simulink model "controller"  (R2018b)
settings: Solver=FixedStepAuto  StartTime=0.0  StopTime=15  FixedStep=0.005  RelTol=1e-3
settings Model: NumberOfSteps=50  Creator=XLIYAN  LastModifiedBy=XLIYAN
settings DebuggingCC: VectorMatrixConversionMsg=warning  UnderSpecifiedDimensionMsg=warning

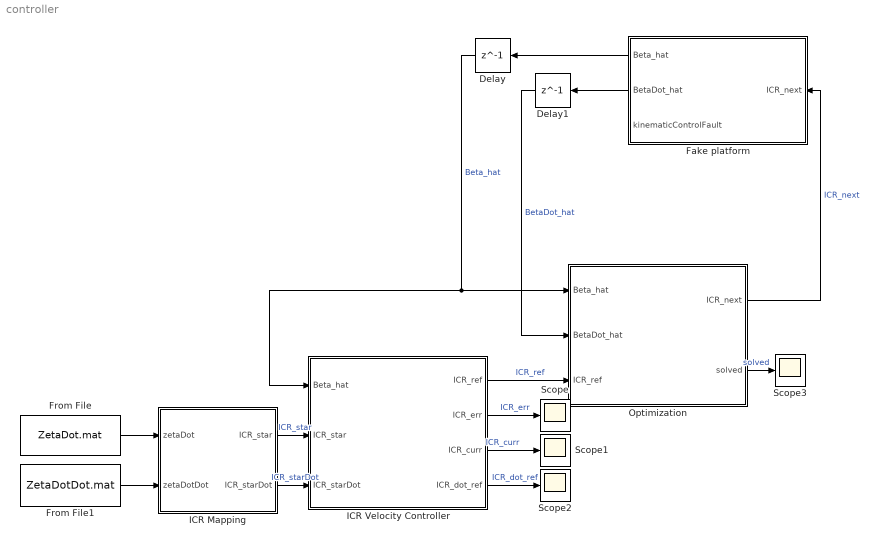
== system controller ==
  Delay : Delay  DelayLength=1  InitialCondition=[0,0,0,0]  InputProcessing=Inherited  SampleTime=0.005
  Delay1 : Delay  DelayLength=1  InitialCondition=[0,0,0,0]  InputProcessing=Inherited  SampleTime=0.005
  Fake platform : MATLAB Function  TreatAsAtomicUnit=on
  From File : FromFile  FileName=ZetaDot.mat  SampleTime=0
  From File1 : FromFile  FileName=ZetaDotDot.mat  SampleTime=0
  ICR Mapping : MATLAB Function  TreatAsAtomicUnit=on
  ICR Velocity Controller : MATLAB Function  TreatAsAtomicUnit=on
  Optimization : MATLAB Function  TreatAsAtomicUnit=on
  Scope{,1..3} (4 alike) : Scope
  wires:
  From File/1 -> ICR Mapping/1(zetaDot)
  From File1/1 -> ICR Mapping/2(zetaDotDot)
  ICR Mapping/1(ICR_star) -> ICR Velocity Controller/2(ICR_star)  "ICR_star"
  ICR Mapping/2(ICR_starDot) -> ICR Velocity Controller/3(ICR_starDot)  "ICR_starDot"
  ICR Velocity Controller/1(ICR_ref) -> Optimization/3(ICR_ref)  "ICR_ref"
  Fake platform/1(Beta_hat) -> Delay/1
  Delay/1 -> ICR Velocity Controller/1(Beta_hat), Optimization/1(Beta_hat)  "Beta_hat"
  Fake platform/2(BetaDot_hat) -> Delay1/1
  Delay1/1 -> Optimization/2(BetaDot_hat)  "BetaDot_hat"
  Optimization/1(ICR_next) -> Fake platform/1(ICR_next)  "ICR_next"
  ICR Velocity Controller/2(ICR_err) -> Scope/1  "ICR_err"
  ICR Velocity Controller/3(ICR_curr) -> Scope1/1  "ICR_curr"
  ICR Velocity Controller/4(ICR_dot_ref) -> Scope2/1  "ICR_dot_ref"
  Optimization/2(solved) -> Scope3/1  "solved"

== matlab function controller/ICR Velocity Controller ==
  data: Beta_hat input; ICR_star input; ICR_ref output; ICR_starDot input; ICR_err output; ICR_curr output; ICR_dot_ref output
function [ICR_ref,ICR_err,ICR_curr,ICR_dot_ref] = ICR_vel_Controller(Beta_hat, ICR_star, ICR_starDot)

vehicle.length = 0.526;  % Vehicle length
vehicle.width = 0.526;   % Vehicle width
wheel.radius = 0.084; %
wheel.offcentre = 0.0; %
a = vehicle.width/2;
b = vehicle.length/2;
rw = wheel.radius;
hx = b;
hy = a;
d = wheel.offcentre;

hx1 = hx;
hx2 = hx;
hx3 = -hx;
hx4 = -hx;

hy1 = -hy;
hy2 =  hy;
hy3 =  hy;
hy4 = -hy;

hx =[hx1, hx2, hx3, hx4];
hy =[hy1, hy2, hy3, hy4];

P_gain=3.7;
deltaT=0.005;
index=[1,4];
max_diff=0;
betaThreshold=0.0236;
R_max = 10;
ICR_curr=[0,R_max];
for i=1:4
    for j=i:4
        if(abs(Beta_hat(i)-Beta_hat(j)>max_diff))
            max_diff = max(abs(Beta_hat(i)-Beta_hat(j)),max_diff);
            index=[i,j];
        end
    end
end


if(abs(Beta_hat(index(1)))<betaThreshold)
    ICR_curr(2) = R_max*cos(Beta_hat(index(1)));
    ICR_curr(1) = R_max*sin(Beta_hat(index(1)));
else
    ICR_curr(2) = (hx(index(1))-hx(index(2))+hy(index(1))*tan(Beta_hat(index(1)))-hy(index(2))*tan(Beta_hat(index(2))))/(tan(Beta_hat(index(1)))-tan(Beta_hat(index(2))));
    ICR_curr(1) = hx(index(1))-tan(Beta_hat(index(1)))*(ICR_curr(2)-hy(index(1)));
end

ICR_err=ICR_star-ICR_curr;
ICR_dot_ref=ICR_starDot + P_gain*ICR_err;
ICR_ref = ICR_curr + ICR_dot_ref*deltaT;

== matlab function controller/ICR Mapping ==
  data: zetaDot input; ICR_star output; zetaDotDot input; ICR_starDot output
function [ICR_star, ICR_starDot] = mappingICR(zetaDot, zetaDotDot)
R_max = 10;
% V_max = 10;
delta1 = 1e-9;
deltaT=0.005;
persistent previousICRstar;
if isempty(previousICRstar)
    previousICRstar = [0,0];
end

ICR_X_star = R_max * tanh(-zetaDot(2)/(zetaDot(3) + delta1*sign(1-any(zetaDot(3),2)+zetaDot(3)))/R_max);
ICR_Y_star = R_max * tanh(zetaDot(1)/(zetaDot(3) + delta1*sign(1-any(zetaDot(3),2)+zetaDot(3)))/R_max);
ICR_star=[ICR_X_star,ICR_Y_star];
% ICR_X_starDot = V_max * tanh((zetaDotDot(3)*zetaDot(2)-zetaDotDot(2)*zetaDot(3))/(zetaDot(3)^2+delta1)/V_max);
% %ICR_Y_starDot = V_max * tanh((zetaDotDot(1)*zetaDot(3)-zetaDotDot(3)*zetaDot(1))/(zetaDot(3)^2+delta1)/V_max);
% ICR_Y_starDot=0;

%backward finite difference
ICR_starDot=(ICR_star-previousICRstar)/deltaT;
previousICRstar=ICR_star;

== matlab function controller/Optimization ==
  data: Beta_hat input; ICR_next output; BetaDot_hat input; ICR_ref input; solved output
function [ICR_next,solved] = Optimization(Beta_hat, BetaDot_hat, ICR_ref)

solved=0;
deltaT=0.005;
%% Parameters of mobiler robot from the paper

hx1 = 0.263;
hx2 = 0.263; 
hx3 = -0.263;
hx4 = -0.263;

hy1 = -0.263;
hy2 = 0.263;
hy3 = 0.263;
hy4 = -0.263;

hxi =[hx1, hx2, hx3, hx4];
hyi =[hy1, hy2, hy3, hy4];
h_i=[hxi(1),hyi(1);hxi(2),hyi(2);hxi(3),hyi(3);hxi(4),hyi(4)];


Limit_Betadot = 2;%(rad/s)
Limit_Betadotdot = 25;%(rad/s^2)
Betadot_max_end=zeros(1,4);
Betadot_min_end=zeros(1,4);
Beta_max=zeros(1,4);
Beta_min=zeros(1,4);

%% QP parameters

P = [1,0;0,1];
q = [-ICR_ref(1),-ICR_ref(2)]';

A=zeros(8,2);
b=[Inf;Inf;Inf;Inf;Inf;Inf;Inf;Inf];

x_new=ICR_ref';
u_new=zeros(size(A,1),1);
z_new=zeros(size(A,1),1);

Max_Iterate=1000;
rho=1;
ABSTOL= sqrt(2)*1e-4;
RELTOL= 1e-2;
%compute constraints
for i=1:4
    %Calculate max/min ending velocity in this time interval
    %if BetaDot=0, process it as BetaDot>0
    if(BetaDot_hat(i)<0)
        Betadot_max_end(i)=max((BetaDot_hat(i) - deltaT*Limit_Betadotdot),-Limit_Betadot);
        Betadot_min_end(i)=min((BetaDot_hat(i) + deltaT*Limit_Betadotdot), Limit_Betadot);
    else
        Betadot_max_end(i)=min((BetaDot_hat(i) + deltaT*Limit_Betadotdot), Limit_Betadot);
        Betadot_min_end(i)=max((BetaDot_hat(i) - deltaT*Limit_Betadotdot), -Limit_Betadot);
    end
    
    Beta_max(i)=Beta_hat(i)+ deltaT*Betadot_max_end(i);
    Beta_min(i)=Beta_hat(i)+ deltaT*Betadot_min_end(i);
    
    
    if((Beta_max(i)>pi)||(Beta_max(i)<0))
        if(BetaDot_hat(i)<0)
            A(2*i-1,:)=[-cot(Beta_max(i)),-1];
            b(2*i-1)=[-cot(Beta_max(i)),-1]*h_i(i,:)';
        else
            A(2*i-1,:)=[cot(Beta_max(i)),1];
            b(2*i-1)=[cot(Beta_max(i)),1]*h_i(i,:)';
        end
        
    else
        if(BetaDot_hat(i)<0)
            A(2*i-1,:)=[cot(Beta_max(i)),1];
            b(2*i-1)=[cot(Beta_max(i)),1]*h_i(i,:)';
        else
            A(2*i-1,:)=[-cot(Beta_max(i)),-1];
            b(2*i-1)=[-cot(Beta_max(i)),-1]*h_i(i,:)';
        end
        
    end
    
    
    
    if((Beta_min(i)>pi)||(Beta_min(i)<0))
        if(BetaDot_hat(i)<0)
            A(2*i,:)=[cot(Beta_min(i)),1];
            b(2*i)=[cot(Beta_min(i)),1]*h_i(i,:)';
        else
            A(2*i,:)=[-cot(Beta_min(i)),-1];
            b(2*i)=[-cot(Beta_min(i)),-1]*h_i(i,:)';
        end
        
    else
        if(BetaDot_hat(i)<0)
            A(2*i,:)=[-cot(Beta_min(i)),-1];
            b(2*i)=[-cot(Beta_min(i)),-1]*h_i(i,:)';
        else
            A(2*i,:)=[cot(Beta_min(i)),1];
            b(2*i)=[cot(Beta_min(i)),1]*h_i(i,:)';
        end
    end
    
end

%%debugging and plot section
% if(k==510)
%     r = ICR_X_ref(k)^2+ICR_Y_ref(k)^2;
% end

%%feasibility check
for i=1:8
    value=A(i,:)*ICR_ref';
    if(value<b(i))
        feasibility=1;
    else
        feasibility=0;
        break;
    end
end
if(feasibility==0)
    N = -(P + rho*(A'*A));
    N2 = N\(rho*A');
    N1 = N\(q - rho*A'*b);
%Solve QP
    for k=1:Max_Iterate
    %x-update
    x_new=N1 + N2*(z_new + u_new);
    %z-update
    z_old=z_new;
    z_new = max(0, -A*x_new - u_new + b);
    %z_new=func_projection(x_new+u_new,A,b);
    
    %u-update
    u_new=u_new+(A*x_new - b + z_new);
    
    %termination check
    primal_residual=norm(A*x_new - b + z_new);
    dual_residual=norm(-rho*(z_new-z_old));
    eps_pri= ABSTOL + RELTOL*max(norm(x_new), norm(-z_new));
    eps_dual= ABSTOL + RELTOL*norm(rho*u_new);
    if(primal_residual<eps_pri && dual_residual<eps_dual)
        solved=5;
        break;
    end
    solved=-5;
    end
    
    
    ICR_next=[x_new(1),x_new(2)];
    
else
    %ICR_ref is inside of feasible set, no need to optimize
    ICR_next=[ICR_ref(1),ICR_ref(2)];
    solved=1;
end
%  XP=-1:0.01:1;
% % 
%  figure(1)
%  for i=1:8
%     if(A(i,2)>0)
%         YP=-A(i,1)*XP + b(i);
%     else
%         YP=A(i,1)*XP - b(i);
%     end
% %     %             YP=-cot(Beta(i))*XP + cot(Beta(i))*h_i(i,1)+h_i(i,2);
%      plot(XP,YP);
%      hold on;
%  end
% scatter(h_i(1,1),h_i(1,2));
% hold on;
% scatter(h_i(2,1),h_i(2,2));
% hold on;
% scatter(h_i(3,1),h_i(3,2));
% hold on;
% scatter(h_i(4,1),h_i(4,2));
% hold on;
% scatter(ICR_ref(1),ICR_ref(2),"filled");
% hold on;
% 
% scatter(ICR_next(1),ICR_next(2));

== matlab function controller/Fake platform ==
  data: Beta_hat output; ICR_next input; BetaDot_hat output; kinematicControlFault output
function [Beta_hat,  BetaDot_hat, kinematicControlFault] = FeedbackModel(ICR_next)
% File initialization

persistent initialPositionIsSet;
if isempty(initialPositionIsSet)
    rng('shuffle');
    initialPositionIsSet = false;
end

persistent Beta_curr;
if isempty(Beta_curr)
    Beta_curr = zeros(4,1);
end

persistent fault;
if isempty(fault)
    fault = false;
end
vehicle.length = 0.526;  % Vehicle length
vehicle.width = 0.526;   % Vehicle width
wheel.radius = 0.084; %
wheel.offcentre = 0.0; %
a = vehicle.width/2;
b = vehicle.length/2;
rw = wheel.radius;
hx = b;
hy = a;
d = wheel.offcentre;

hx1 = hx;
hx2 = hx;
hx3 = -hx;
hx4 = -hx;

hy1 = -hy;
hy2 =  hy;
hy3 =  hy;
hy4 = -hy;

hxi =[hx1, hx2, hx3, hx4];
hyi =[hy1, hy2, hy3, hy4];

Limit_Betadot = 2;%(rad/s)
Limit_Betadotdot = 25;%(rad/s^2)
deltaT = 0.005;
delta1 = 1e-9;

Beta_hat = zeros(4,1);
BetaDot_hat = zeros(4,1);




% Pose store in glboal coordinate system
%if  ~isnan(xdotB) && ~isnan(ydotB) && ~isnan(thetadotB) && ~isnan(xdotdotB) && ~isnan(ydotdotB) && ~isnan(thetadotdotB)
if  ~isnan(ICR_next(1)) && ~isnan(ICR_next(2))    

        for i = 1:4
            
            Beta_hat(i) = atan2((ICR_next(2)-hyi(i)),(ICR_next(1)-hxi(i)))-0.5*pi;
            %Beta_hat(i) = atan((ICR_next(1)-hxi(i))/(ICR_next(2)-hyi(i)));
            deltaBeta = Beta_hat(i) - Beta_curr(i);
            noise=Limit_Betadot*deltaT*1e-2*randn;
            if abs(deltaBeta) > (pi + pi/2)
                %jump detected 
                if Beta_curr(i) > 0
                    Beta_hat(i) = -sign(Beta_hat(i))*Beta_hat(i) + 2*pi;
                else
                    Beta_hat(i) = sign(Beta_hat(i))*Beta_hat(i) - 2*pi;           
                end
            elseif abs(deltaBeta) > pi/2
                %jump detected 
                if Beta_curr(i) > 0
                    Beta_hat(i) = Beta_hat(i) + pi;              
                else
                    Beta_hat(i) = Beta_hat(i) - pi;                    
                end
                %otherwise leave beta unchanged     
            end
            %introduce noise to simulate sensor feedback
            Beta_hat(i)=Beta_hat(i) + noise;

            %calculate betaDot
            if deltaBeta<(2*Limit_Betadot*deltaT - 2*pi)
                BetaDot_hat(i)=(deltaBeta + noise + 2*pi)/deltaT;
            elseif deltaBeta>(2*pi - 2*Limit_Betadot*deltaT)
                BetaDot_hat(i)=(deltaBeta + noise - 2*pi)/deltaT;
            else
                BetaDot_hat(i)=(deltaBeta+ noise)/deltaT;
            end
        end

%         if ~initialPositionIsSet
%             previousBeta = Beta_hat;
%             initialPositionIsSet = true;
%         end
        
        
         Beta_curr = Beta_hat;
    
else
    fault = true;
end
% 
% if isnan(Beta(1)) || isnan(Betaidot(1)) || isnan(Phi_dot(1)) ||...
%         isnan(Beta(2)) || isnan(Betaidot(2)) || isnan(Phi_dot(2)) ||...
%         isnan(Beta(3)) || isnan(Betaidot(3)) || isnan(Phi_dot(3)) ||...
%         isnan(Beta(4)) || isnan(Betaidot(4)) || isnan(Phi_dot(4))
%     fault = true;
%     initialPoseBus.SteerMotor1Position = 0;
%     initialPoseBus.SteerMotor2Position = 0;
%     initialPoseBus.SteerMotor3Position = 0;
%     initialPoseBus.SteerMotor4Position = 0;
% else
%     initialPoseBus.SteerMotor1Position = Beta(2);
%     initialPoseBus.SteerMotor2Position = Beta(1);
%     initialPoseBus.SteerMotor3Position = Beta(4);
%     initialPoseBus.SteerMotor4Position = Beta(3);
% end



kinematicControlFault = fault;
